simulink subsystem "Nitrous_Tank"  (R2020b)
settings: Solver=VariableStepAuto  StartTime=0.0  StopTime=10.0  RelTol=1e-3
model mask{nitrousFluidPropsTable=sim.nitrousFluidTable, nitrousLiqConCrossSection=3.8485e-05, nitrousVapConCrossSection=2e-5, nitrousTankVol=0.0141, initialTankPressure=60e5, initialLiqMassFraction=0.7}
  mask prompts: nitrousFluidPropsTable "The nitrous oxide two phase fluid data table"; nitrousLiqConCrossSection "Liquid port cross section in m^2"; nitrousVapConCrossSection "Vapour port cross section in m^2"; nitrousTankVol "Tank Volume in m^3"; initialTankPressure "Tank start pressure in Pa"; initialLiqMassFraction "Fraction of the nitrous in the tank which starts out liquid (By mass)"
libraries: fl_lib x12, nesl_utility x5, SimscapeFluids_lib x1
settings Model: Creator=Edward  LastModifiedBy=luc

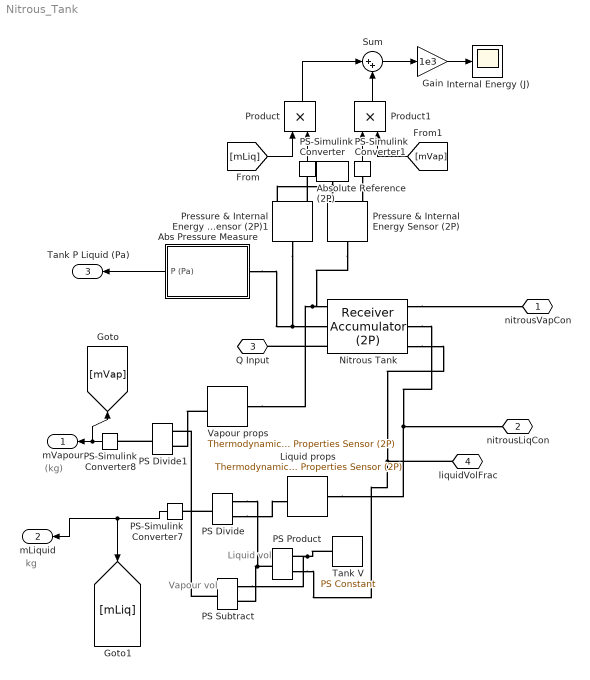
== system Nitrous_Tank ==
  note: kg
  note: (kg)
  note: Vapour vol
  note: Liquid vol
  Abs Pressure Measure : Subsystem
  Absolute Reference (2P) : fl_lib/Two-Phase Fluid/Elements/Absolute Reference (2P)
      settings: SourceProductBaseCode=SS
  Gain : Gain  Gain=1e3
  "Internal Energy (J) " : Scope
  Liquid props : fl_lib/Two-Phase Fluid/Sensors/Thermodynamic Properties Sensor (2P)
      settings: SourceProductBaseCode=SS  InternalSimscapePortConfiguration="{\"Bottom\":[],\"Left\":[{\"id\":\"A\",\"label\":\"A\",\"type\":\"foundation.two_phase_fluid.two_phase_fluid\"}],\"Right\":[{\"id\":\"T\",\"label\":\"T\",\"type\":\"output\"},{\"id\":\"H\",\"label\":\"h\",\"type\":\"output\"},{\"id\":\"V\",\"label\":\"v\",\"type\":\"output\"},{\"id\":\"S\",\"label\":\"s\",\"type\":\"output\"}],\"Top\":[]}"
  Nitrous Tank : SimscapeFluids_lib/Two-Phase Fluid/Tanks & Accumulators/Receiver Accumulator (2P)  volume=nitrousTankVol m^3  area_AV=2e-5 m^2  area_BV=nitrousVapConCrossSection m^2  area_AL=2e-5 m^2  area_BL=nitrousLiqConCrossSection m^2  V_frac_error=simscape.enum.assert.action.none  V_frac_min=0.05  V_frac_max=0.95  V_frac_smooth=0.04  p_crit_error=simscape.enum.assert.action.error  hc_vap=20 W/(m^2 * K)  hc_liq=100 W/(m^2 * K)  surface_area=6 m^2  receiver_accumulator_energy_spec=fluids.two_phase_fluid.enum.receiver_accumulator_energy_spec.mass_fraction  p_init=initialTankPressure Pa  T_init=293.15 K  M_frac_init=initialLiqMassFraction  V_frac_init=0.55  h_init=1500 kJ/kg  u_init=1500 kJ/kg  tau_vap_cond=0.1 s
      settings: SourceProductBaseCode=SH  InternalSimscapePortConfiguration="{\"Bottom\":[],\"Left\":[{\"id\":\"AV\",\"label\":\"AV\",\"type\":\"foundation.two_phase_fluid.two_phase_fluid\"},{\"id\":\"AL\",\"label\":\"AL\",\"type\":\"foundation.two_phase_fluid.two_phase_fluid\"},{\"id\":\"H\",\"label\":\"H\",\"type\":\"foundation.thermal.thermal\"}],\"Right\":[{\"id\":\"BV\",\"label\":\"BV\",\"type\":\"foundation.two_phase_fluid.two_phase_fluid\"},{\"id\":\"BL\",\"label\":\"BL\",\"type\":\"foundation.two_phase_fluid.two_phase_fluid\"},{\"id\":\"L\",\"label\":\"L\",\"type\":\"output\"}],\"Top\":[]}"
  PS Divide : fl_lib/Physical Signals/Functions/PS Divide
      settings: SourceProductBaseCode=SS
  PS Divide1 : fl_lib/Physical Signals/Functions/PS Divide
      settings: SourceProductBaseCode=SS
  PS Product : fl_lib/Physical Signals/Functions/PS Product
  PS Subtract : fl_lib/Physical Signals/Functions/PS Subtract
  PS-Simulink Converter{,1,7..8} (4 alike) : nesl_utility/PS-Simulink Converter  PhysicalDomain=network_engine_domain  SubClassName=ps_output  LeftPortType=input  RightPortType=output  PseudoPeriodic=off  Frequencies=[]  Unit=inherit  AffineConversion=off
  Pressure & Internal Energy Sensor (2P) : fl_lib/Two-Phase Fluid/Sensors/Pressure & Internal Energy Sensor (2P)
      settings: SourceProductBaseCode=SS  InternalSimscapePortConfiguration="{\"Bottom\":[],\"Left\":[{\"id\":\"A\",\"label\":\"A\",\"type\":\"foundation.two_phase_fluid.two_phase_fluid\"}],\"Right\":[{\"id\":\"B\",\"label\":\"B\",\"type\":\"foundation.two_phase_fluid.two_phase_fluid\"},{\"id\":\"P\",\"label\":\"P\",\"type\":\"output\"},{\"id\":\"U\",\"label\":\"U\",\"type\":\"output\"}],\"Top\":[]}"
  Pressure & Internal Energy Sensor (2P)1 : fl_lib/Two-Phase Fluid/Sensors/Pressure & Internal Energy Sensor (2P)
      settings: SourceProductBaseCode=SS  InternalSimscapePortConfiguration="{\"Bottom\":[],\"Left\":[{\"id\":\"A\",\"label\":\"A\",\"type\":\"foundation.two_phase_fluid.two_phase_fluid\"}],\"Right\":[{\"id\":\"B\",\"label\":\"B\",\"type\":\"foundation.two_phase_fluid.two_phase_fluid\"},{\"id\":\"P\",\"label\":\"P\",\"type\":\"output\"},{\"id\":\"U\",\"label\":\"U\",\"type\":\"output\"}],\"Top\":[]}"
  Product : Product
  Product1 : Product
  Sum : Sum  Inputs=|++
  "Tank V " : fl_lib/Physical Signals/Sources/PS Constant  constant=sim.runTank.volume m^3
  Vapour props : fl_lib/Two-Phase Fluid/Sensors/Thermodynamic Properties Sensor (2P)
      settings: SourceProductBaseCode=SS  InternalSimscapePortConfiguration="{\"Bottom\":[],\"Left\":[{\"id\":\"A\",\"label\":\"A\",\"type\":\"foundation.two_phase_fluid.two_phase_fluid\"}],\"Right\":[{\"id\":\"T\",\"label\":\"T\",\"type\":\"output\"},{\"id\":\"H\",\"label\":\"h\",\"type\":\"output\"},{\"id\":\"V\",\"label\":\"v\",\"type\":\"output\"},{\"id\":\"S\",\"label\":\"s\",\"type\":\"output\"}],\"Top\":[]}"
  nitrousVapCon : PMIOPort  Side=Right
  nitrousLiqCon : PMIOPort  Port=2  Side=Right
  Q Input : PMIOPort  Port=3  Side=Left
  liquidVolFrac : PMIOPort  Port=4  Side=Right
  mVapour : Outport
  mLiquid : Outport  Port=2
  Tank P Liquid (Pa) : Outport  Port=3
  wires:
  PS-Simulink Converter7/1 -> [mLiq], mLiquid/1
  PS-Simulink Converter8/1 -> mVapour/1, [mVap]
  Abs Pressure Measure/1(P (Pa)) -> Tank P Liquid (Pa)/1
  PS-Simulink Converter/1 -> Product/2
  [mLiq] -> Product/1
  PS-Simulink Converter1/1 -> Product1/1
  [mVap] -> Product1/2
  Product1/1 -> Sum/2
  Product/1 -> Sum/1
  Sum/1 -> Gain/1
  Gain/1 -> "Internal Energy (J) "/1
  connections:
  Nitrous Tank/RConn2 -- Liquid props/LConn1 -- nitrousLiqCon/RConn1
  PS Product/LConn2 -- Nitrous Tank/RConn3 -- liquidVolFrac/RConn1
  PS Divide/LConn1 -- PS Product/RConn1 -- PS Subtract/LConn2
  Pressure & Internal Energy Sensor (2P)/LConn1 -- Vapour props/LConn1 -- Nitrous Tank/LConn1
  PS Subtract/LConn1 -- "Tank V "/RConn1 -- PS Product/LConn1
  Pressure & Internal Energy Sensor (2P)1/LConn1 -- Abs Pressure Measure/LConn1 -- Nitrous Tank/LConn2
  Pressure & Internal Energy Sensor (2P)1/RConn1 -- Absolute Reference (2P)/LConn1 -- Pressure & Internal Energy Sensor (2P)/RConn1
  Nitrous Tank/RConn1 -- nitrousVapCon/RConn1
  Vapour props/RConn3 -- PS Divide1/LConn2
  PS Divide/RConn1 -- PS-Simulink Converter7/LConn1
  PS Subtract/RConn1 -- PS Divide1/LConn1
  PS Divide/LConn2 -- Liquid props/RConn3
  PS Divide1/RConn1 -- PS-Simulink Converter8/LConn1
  Nitrous Tank/LConn3 -- Q Input/RConn1
  Pressure & Internal Energy Sensor (2P)1/RConn3 -- PS-Simulink Converter/LConn1
  PS-Simulink Converter1/LConn1 -- Pressure & Internal Energy Sensor (2P)/RConn3

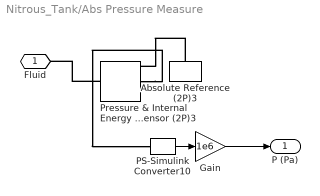
== system Nitrous_Tank/Abs Pressure Measure ==
  Absolute Reference (2P)3 : fl_lib/Two-Phase Fluid/Elements/Absolute Reference (2P)
      settings: SourceProductBaseCode=SS
  Gain : Gain  Gain=1e6
  PS-Simulink Converter10 : nesl_utility/PS-Simulink Converter  PhysicalDomain=network_engine_domain  SubClassName=ps_output  LeftPortType=input  RightPortType=output  PseudoPeriodic=off  Frequencies=[]  Unit=inherit  AffineConversion=off
  Pressure & Internal Energy Sensor (2P)3 : fl_lib/Two-Phase Fluid/Sensors/Pressure & Internal Energy Sensor (2P)
      settings: SourceProductBaseCode=SS  InternalSimscapePortConfiguration="{\"Bottom\":[],\"Left\":[{\"id\":\"A\",\"label\":\"A\",\"type\":\"foundation.two_phase_fluid.two_phase_fluid\"}],\"Right\":[{\"id\":\"B\",\"label\":\"B\",\"type\":\"foundation.two_phase_fluid.two_phase_fluid\"},{\"id\":\"P\",\"label\":\"P\",\"type\":\"output\"},{\"id\":\"U\",\"label\":\"U\",\"type\":\"output\"}],\"Top\":[]}"
  Fluid : PMIOPort  Side=Left
  P (Pa) : Outport
  wires:
  Gain/1 -> P (Pa)/1
  PS-Simulink Converter10/1 -> Gain/1
  connections:
  Pressure & Internal Energy Sensor (2P)3/LConn1 -- Fluid/RConn1
  Pressure & Internal Energy Sensor (2P)3/RConn2 -- PS-Simulink Converter10/LConn1
  Absolute Reference (2P)3/LConn1 -- Pressure & Internal Energy Sensor (2P)3/RConn1
